simulink library "SPART_Lib"  (R2016b)
settings: Solver=ode45  StartTime=0.0  StopTime=10.0  RelTol=1e-3  EnableMultiTasking=on
undefined symbols (not defined in the file): n, Newton, q00, q0dot0, qm0, Raphson, robot, T_Ln_EE
libraries: SPART_Lib x3, dspinverses x1
settings Model: Creator=Josep  LastModifiedBy=Josep
settings DataIOCC: LimitDataPoints=on  SaveFormat=Array
settings OptimizationCC: LifeSpan=inf
settings DebuggingCC: AllowSymbolicDim=off  SFUnexpectedBacktrackingDiag=warning  SFNoUnconditionalDefaultTransitionDiag=warning  SFExecutionAtInitializationDiag=none
settings HardwareCC: ProdBitPerPointer=32  ProdBitPerSizeT=32  ProdBitPerPtrDiffT=32  ProdLargestAtomicFloat=None  ProdIntDivRoundTo=Undefined  ProdEndianess=Unspecified  ProdWordSize=32  ProdHWDeviceType=32-bit Generic
settings ModelReferenceCC: PropagateSignalLabelsOutOfModel=off
settings GRTTargetCC: TargetLangStandard=C89/C90 (ANSI)  GeneratePreprocessorConditionals=Disable all
settings ConfigComp: CovMetricSettings=dw  CovHtmlReporting=on  CovSaveCumulativeToWorkspaceVar=on  CovSaveSingleToWorkspaceVar=on  CovExternalEMLEnable=off

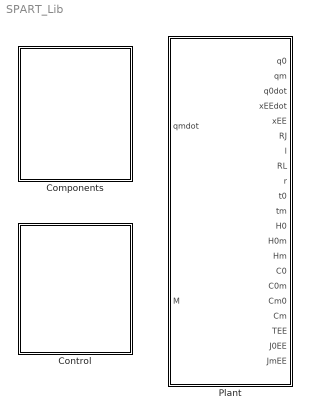
== system SPART_Lib ==
  Components : Subsystem
  Control : Subsystem
  Plant : Subsystem  TreatAsAtomicUnit=on
      settings: MinAlgLoopOccurrences=on

== system SPART_Lib/Components ==
  Base Reaction : Subsystem
  EndEffector : Subsystem
  Jstar : Subsystem
  Matrices : Subsystem

== system SPART_Lib/Control ==
  Base Control : Subsystem
  Desired-Reaction-Maneuver : Subsystem  mask{xdot_I=[1:6], q0dot_I=[1:6]}
      mask prompts: xdot_I "xdot - Indices"; q0dot_I "q0dot - Indices"
      mask help: Desired-Reaction-Maneuver
      settings: MinAlgLoopOccurrences=on
  "Resolved-Motion-Rate " : Subsystem
      settings: MinAlgLoopOccurrences=on
  Resolved-Motion-Rate Minimize Floating Kinematic Energy : Subsystem
      settings: MinAlgLoopOccurrences=on

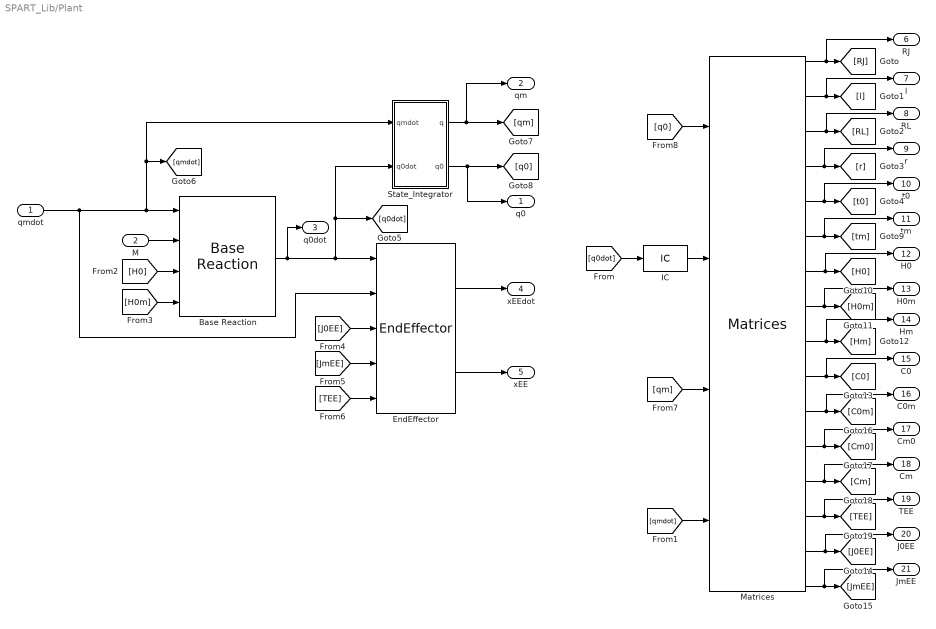
== system SPART_Lib/Plant ==
  qmdot : Inport
  M : Inport  Port=2
  Base Reaction : SPART_Lib/Components/Base Reaction
  EndEffector : SPART_Lib/Components/EndEffector
  IC : InitialCondition  Value=q0dot0
  Matrices : SPART_Lib/Components/Matrices
  State_Integrator : Subsystem
  "q0 " : Outport
  qm : Outport  Port=2
  "q0dot " : Outport  Port=3
  xEEdot : Outport  Port=4
  xEE : Outport  Port=5
  RJ : Outport  Port=6
  l : Outport  Port=7
  RL : Outport  Port=8
  r : Outport  Port=9
  t0 : Outport  Port=10
  "tm " : Outport  Port=11
  "H0 " : Outport  Port=12
  "H0m " : Outport  Port=13
  "Hm " : Outport  Port=14
  "C0 " : Outport  Port=15
  "C0m " : Outport  Port=16
  "Cm0 " : Outport  Port=17
  "Cm " : Outport  Port=18
  TEE : Outport  Port=19
  "J0EE " : Outport  Port=20
  JmEE : Outport  Port=21
  wires:
  [q0dot] -> IC/1
  IC/1 -> Matrices/2
  [q0] -> Matrices/1
  [qm] -> Matrices/3
  [qmdot] -> Matrices/4
  Matrices/1 -> RJ/1, [RJ]
  [H0] -> Base Reaction/3
  [H0m] -> Base Reaction/4
  [J0EE] -> EndEffector/3
  [JmEE] -> EndEffector/4
  [TEE] -> EndEffector/5
  Base Reaction/1 -> "q0dot "/1, EndEffector/1, State_Integrator/2(q0dot), [q0dot]
  qmdot/1 -> EndEffector/2, Base Reaction/1, [qmdot], State_Integrator/1(qmdot)
  M/1 -> Base Reaction/2
  State_Integrator/1(q) -> qm/1, [qm]
  State_Integrator/2(q0) -> "q0 "/1, [q0]
  Matrices/2 -> l/1, [l]
  Matrices/3 -> [RL], RL/1
  Matrices/4 -> r/1, [r]
  Matrices/5 -> t0/1, [t0]
  EndEffector/2 -> xEE/1
  EndEffector/1 -> xEEdot/1
  Matrices/6 -> "tm "/1, [tm]
  Matrices/7 -> "H0 "/1, [H0]
  Matrices/8 -> "H0m "/1, [H0m]
  Matrices/9 -> "Hm "/1, [Hm]
  Matrices/10 -> "C0 "/1, [C0]
  Matrices/11 -> [C0m], "C0m "/1
  Matrices/12 -> "Cm0 "/1, [Cm0]
  Matrices/13 -> "Cm "/1, [Cm]
  Matrices/14 -> TEE/1, [TEE]
  Matrices/15 -> "J0EE "/1, [J0EE]
  Matrices/16 -> JmEE/1, [JmEE]

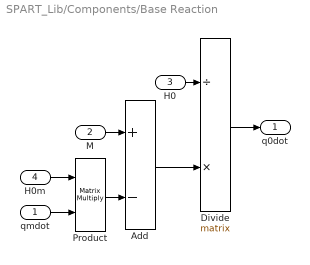
== system SPART_Lib/Components/Base Reaction ==
  qmdot : Inport
  M : Inport  Port=2
  H0 : Inport  Port=3
  H0m : Inport  Port=4
  Add : Sum  Inputs=+-
  Divide : Product  Inputs=/*  Multiplication=Matrix(*)
  Product : Product  Multiplication=Matrix(*)
  q0dot : Outport
  wires:
  Divide/1 -> q0dot/1
  H0/1 -> Divide/1
  M/1 -> Add/1
  Add/1 -> Divide/2
  Product/1 -> Add/2
  H0m/1 -> Product/1
  qmdot/1 -> Product/2

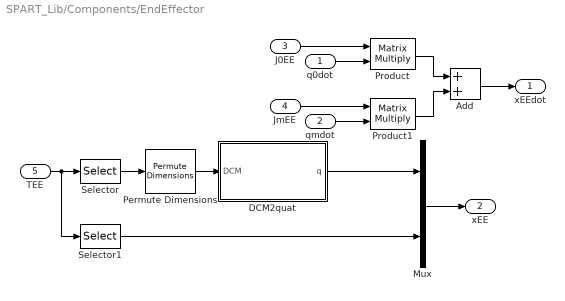
== system SPART_Lib/Components/EndEffector ==
  "q0dot " : Inport
  qmdot : Inport  Port=2
  J0EE : Inport  Port=3
  JmEE : Inport  Port=4
  TEE : Inport  Port=5
  Add : Sum
  DCM2quat : MATLAB Function  TreatAsAtomicUnit=on
  Mux : Mux  Inputs=2
  Permute Dimensions : PermuteDimensions
  Product : Product  Multiplication=Matrix(*)
  Product1 : Product  Multiplication=Matrix(*)
  Selector : Selector  NumberOfDimensions=2  InputPortWidth=6  IndexOptions=Index vector (dialog),Index vector (dialog)  Indices=[1:3],[1:3]  OutputSizes=1,1
  Selector1 : Selector  NumberOfDimensions=2  InputPortWidth=6  IndexOptions=Index vector (dialog),Index vector (dialog)  Indices=[1:3],[4]  OutputSizes=1,1
  xEEdot : Outport
  xEE : Outport  Port=2
  wires:
  Product/1 -> Add/1
  Product1/1 -> Add/2
  Add/1 -> xEEdot/1
  "q0dot "/1 -> Product/2
  qmdot/1 -> Product1/2
  Mux/1 -> xEE/1
  J0EE/1 -> Product/1
  JmEE/1 -> Product1/1
  DCM2quat/1(q) -> Mux/1
  Selector/1 -> Permute Dimensions/1
  TEE/1 -> Selector/1, Selector1/1
  Selector1/1 -> Mux/2
  Permute Dimensions/1 -> DCM2quat/1(DCM)

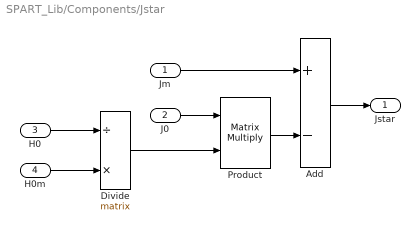
== system SPART_Lib/Components/Jstar ==
  "Jm " : Inport
  J0 : Inport  Port=2
  H0 : Inport  Port=3
  H0m : Inport  Port=4
  Add : Sum  Inputs=+-
  Divide : Product  Inputs=/*  Multiplication=Matrix(*)
  Product : Product  Multiplication=Matrix(*)
  Jstar : Outport
  wires:
  H0m/1 -> Divide/2
  Add/1 -> Jstar/1
  J0/1 -> Product/1
  Divide/1 -> Product/2
  H0/1 -> Divide/1
  Product/1 -> Add/2
  "Jm "/1 -> Add/1

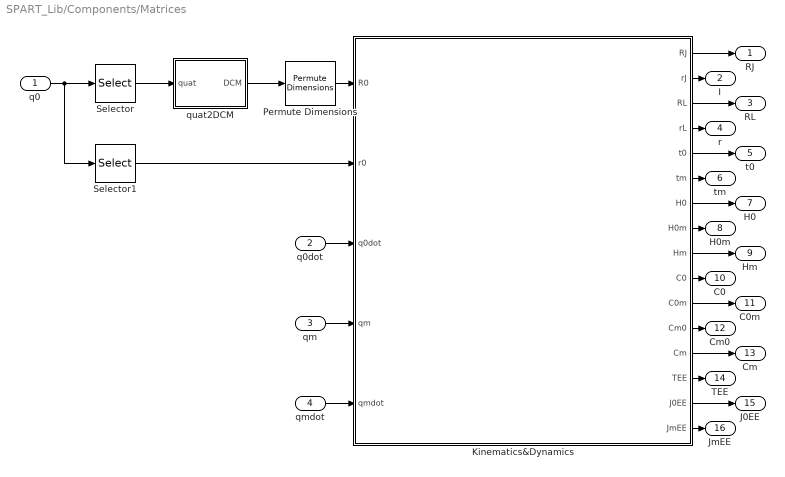
== system SPART_Lib/Components/Matrices ==
  q0 : Inport
  "q0dot " : Inport  Port=2
  qm : Inport  Port=3
  qmdot : Inport  Port=4
  Kinematics&Dynamics : MATLAB Function  TreatAsAtomicUnit=on
  Permute Dimensions : PermuteDimensions
  Selector : Selector  InputPortWidth=7  IndexOptions=Index vector (dialog)  Indices=[1:4]  OutputSizes=1
  Selector1 : Selector  InputPortWidth=7  IndexOptions=Index vector (dialog)  Indices=[5:7]  OutputSizes=1
  quat2DCM : MATLAB Function  TreatAsAtomicUnit=on
  RJ : Outport
  I : Outport  Port=2
  RL : Outport  Port=3
  r : Outport  Port=4
  t0 : Outport  Port=5
  tm : Outport  Port=6
  H0 : Outport  Port=7
  H0m : Outport  Port=8
  Hm : Outport  Port=9
  C0 : Outport  Port=10
  C0m : Outport  Port=11
  Cm0 : Outport  Port=12
  Cm : Outport  Port=13
  TEE : Outport  Port=14
  J0EE : Outport  Port=15
  JmEE : Outport  Port=16
  wires:
  Kinematics&Dynamics/1(RJ) -> RJ/1
  Kinematics&Dynamics/2(rJ) -> I/1
  Kinematics&Dynamics/3(RL) -> RL/1
  Kinematics&Dynamics/4(rL) -> r/1
  Kinematics&Dynamics/5(t0) -> t0/1
  q0/1 -> Selector/1, Selector1/1
  quat2DCM/1(DCM) -> Permute Dimensions/1
  Selector/1 -> quat2DCM/1(quat)
  Kinematics&Dynamics/6(tm) -> tm/1
  Kinematics&Dynamics/7(H0) -> H0/1
  Kinematics&Dynamics/9(Hm) -> Hm/1
  Selector1/1 -> Kinematics&Dynamics/2(r0)
  Permute Dimensions/1 -> Kinematics&Dynamics/1(R0)
  "q0dot "/1 -> Kinematics&Dynamics/3(q0dot)
  qm/1 -> Kinematics&Dynamics/4(qm)
  qmdot/1 -> Kinematics&Dynamics/5(qmdot)
  Kinematics&Dynamics/8(H0m) -> H0m/1
  Kinematics&Dynamics/10(C0) -> C0/1
  Kinematics&Dynamics/12(Cm0) -> Cm0/1
  Kinematics&Dynamics/15(J0EE) -> J0EE/1
  Kinematics&Dynamics/11(C0m) -> C0m/1
  Kinematics&Dynamics/13(Cm) -> Cm/1
  Kinematics&Dynamics/16(JmEE) -> JmEE/1
  Kinematics&Dynamics/14(TEE) -> TEE/1

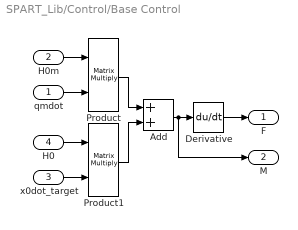
== system SPART_Lib/Control/Base Control ==
  qmdot : Inport
  H0m : Inport  Port=2
  x0dot_target : Inport  Port=3
  H0 : Inport  Port=4
  Add : Sum
  Derivative : Derivative
  Product : Product  Multiplication=Matrix(*)
  Product1 : Product  Multiplication=Matrix(*)
  F : Outport
  M : Outport  Port=2
  wires:
  H0m/1 -> Product/1
  qmdot/1 -> Product/2
  Add/1 -> M/1, Derivative/1
  Product/1 -> Add/1
  Product1/1 -> Add/2
  H0/1 -> Product1/1
  x0dot_target/1 -> Product1/2
  Derivative/1 -> F/1

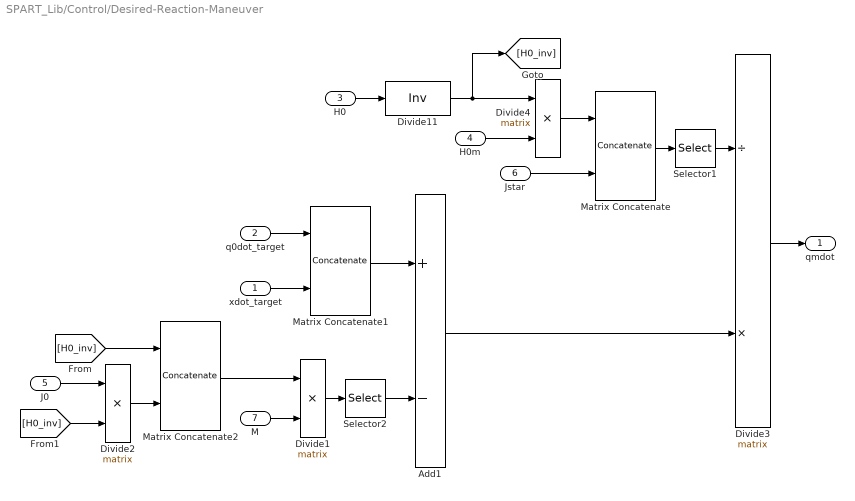
== system SPART_Lib/Control/Desired-Reaction-Maneuver ==
  xdot_target : Inport
  q0dot_target : Inport  Port=2
  H0 : Inport  Port=3
  H0m : Inport  Port=4
  J0 : Inport  Port=5
  Jstar : Inport  Port=6
  M : Inport  Port=7
  Add1 : Sum  Inputs=+-
  Divide1 : Product  Inputs=**  Multiplication=Matrix(*)
  Divide11 : Product  Inputs=/  Multiplication=Matrix(*)
  Divide2 : Product  Inputs=**  Multiplication=Matrix(*)
  Divide3 : Product  Inputs=/*  Multiplication=Matrix(*)
  Divide4 : Product  Inputs=**  Multiplication=Matrix(*)
  Matrix Concatenate : Concatenate  Mode=Multidimensional array
  Matrix Concatenate1 : Concatenate  Mode=Multidimensional array
  Matrix Concatenate2 : Concatenate  Mode=Multidimensional array
  Selector1 : Selector  NumberOfDimensions=2  InputPortWidth=3  IndexOptions=Index vector (dialog),Select all  Indices=[q0dot_I,5+xdot_I],[1:n]  OutputSizes=1,1
  Selector2 : Selector  NumberOfDimensions=2  InputPortWidth=3  IndexOptions=Index vector (dialog),Index vector (dialog)  Indices=[q0dot_I,5+xdot_I],[1]  OutputSizes=1,1
  qmdot : Outport
  wires:
  Divide3/1 -> qmdot/1
  Matrix Concatenate/1 -> Selector1/1
  Divide4/1 -> Matrix Concatenate/1
  H0m/1 -> Divide4/2
  Jstar/1 -> Matrix Concatenate/2
  xdot_target/1 -> Matrix Concatenate1/2
  q0dot_target/1 -> Matrix Concatenate1/1
  Matrix Concatenate1/1 -> Add1/1
  H0/1 -> Divide11/1
  Divide11/1 -> [H0_inv], Divide4/1
  [H0_inv] -> Matrix Concatenate2/1
  Matrix Concatenate2/1 -> Divide1/1
  M/1 -> Divide1/2
  Divide1/1 -> Selector2/1
  Divide2/1 -> Matrix Concatenate2/2
  J0/1 -> Divide2/1
  [H0_inv] -> Divide2/2
  Add1/1 -> Divide3/2
  Selector2/1 -> Add1/2
  Selector1/1 -> Divide3/1

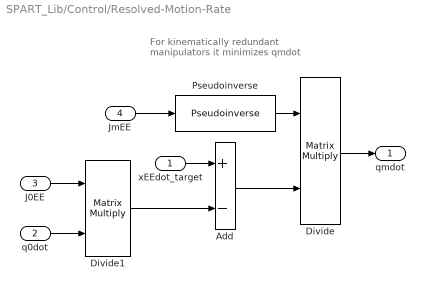
== system SPART_Lib/Control/Resolved-Motion-Rate  ==
  note: For kinematically redundant manipulators it minimizes qmdot
  xEEdot_target : Inport
  q0dot : Inport  Port=2
  J0EE : Inport  Port=3
  JmEE : Inport  Port=4
  Add : Sum  Inputs=+-
  Divide : Product  Inputs=**  Multiplication=Matrix(*)
  Divide1 : Product  Inputs=**  Multiplication=Matrix(*)
  Pseudoinverse : dspinverses/Pseudoinverse  wanterr=off
  qmdot : Outport
  wires:
  Divide/1 -> qmdot/1
  Add/1 -> Divide/2
  Divide1/1 -> Add/2
  J0EE/1 -> Divide1/1
  Pseudoinverse/1 -> Divide/1
  JmEE/1 -> Pseudoinverse/1
  q0dot/1 -> Divide1/2
  xEEdot_target/1 -> Add/1

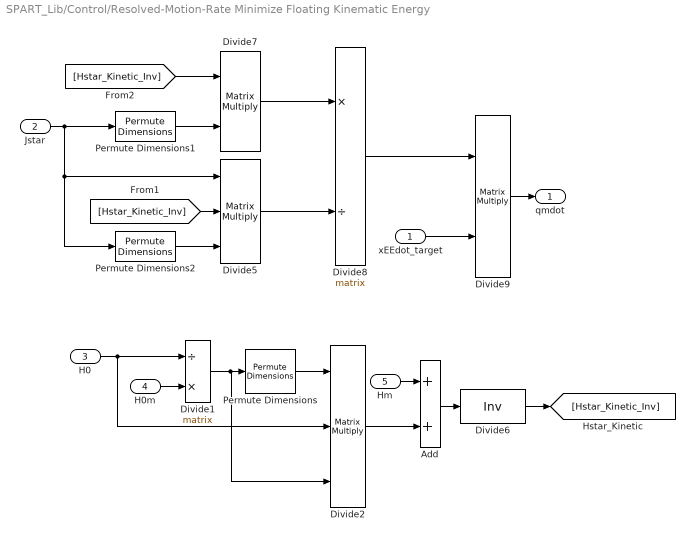
== system SPART_Lib/Control/Resolved-Motion-Rate Minimize Floating Kinematic Energy ==
  xEEdot_target : Inport
  Jstar : Inport  Port=2
  H0 : Inport  Port=3
  H0m : Inport  Port=4
  Hm : Inport  Port=5
  Add : Sum
  Divide1 : Product  Inputs=/*  Multiplication=Matrix(*)
  Divide2 : Product  Inputs=***  Multiplication=Matrix(*)
  Divide5 : Product  Inputs=***  Multiplication=Matrix(*)
  Divide6 : Product  Inputs=/  Multiplication=Matrix(*)
  Divide7 : Product  Inputs=**  Multiplication=Matrix(*)
  Divide8 : Product  Inputs=*/  Multiplication=Matrix(*)
  Divide9 : Product  Inputs=**  Multiplication=Matrix(*)
  Permute Dimensions : PermuteDimensions
  Permute Dimensions1 : PermuteDimensions
  Permute Dimensions2 : PermuteDimensions
  qmdot : Outport
  wires:
  Divide6/1 -> [Hstar_Kinetic_Inv]
  Divide5/1 -> Divide8/2
  Divide9/1 -> qmdot/1
  Divide8/1 -> Divide9/1
  Divide7/1 -> Divide8/1
  Jstar/1 -> Permute Dimensions1/1, Permute Dimensions2/1, Divide5/1
  H0m/1 -> Divide1/2
  Permute Dimensions/1 -> Divide2/1
  Divide1/1 -> Divide2/3, Permute Dimensions/1
  H0/1 -> Divide2/2, Divide1/1
  Divide2/1 -> Add/2
  Hm/1 -> Add/1
  xEEdot_target/1 -> Divide9/2
  [Hstar_Kinetic_Inv] -> Divide7/1
  Permute Dimensions1/1 -> Divide7/2
  [Hstar_Kinetic_Inv] -> Divide5/2
  Add/1 -> Divide6/1
  Permute Dimensions2/1 -> Divide5/3

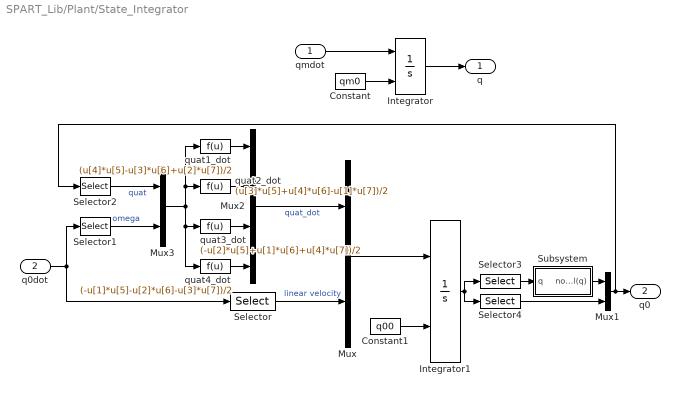
== system SPART_Lib/Plant/State_Integrator ==
  qmdot : Inport
  q0dot : Inport  Port=2
  Constant : Constant  Value=qm0
  Constant1 : Constant  Value=q00
  Integrator : Integrator  InitialConditionSource=external
  Integrator1 : Integrator  InitialConditionSource=external
  Mux : Mux  Inputs=2
  Mux1 : Mux  Inputs=2
  Mux2 : Mux
  Mux3 : Mux  Inputs=2
  Selector : Selector  InputPortWidth=6  IndexOptions=Index vector (dialog)  Indices=[4:6]  OutputSizes=1
  Selector1 : Selector  InputPortWidth=6  IndexOptions=Index vector (dialog)  Indices=[1:3]  OutputSizes=1
  Selector2 : Selector  InputPortWidth=7  IndexOptions=Index vector (dialog)  Indices=[1:4]  OutputSizes=1
  Selector3 : Selector  InputPortWidth=7  IndexOptions=Index vector (dialog)  Indices=[1:4]  OutputSizes=1
  Selector4 : Selector  InputPortWidth=7  IndexOptions=Index vector (dialog)  Indices=[5:7]  OutputSizes=1
  Subsystem : Subsystem
  quat1_dot : Fcn  Expr=(u[4]*u[5]-u[3]*u[6]+u[2]*u[7])/2
  quat2_dot : Fcn  Expr=(u[3]*u[5]+u[4]*u[6]-u[1]*u[7])/2
  quat3_dot : Fcn  Expr=(-u[2]*u[5]+u[1]*u[6]+u[4]*u[7])/2
  quat4_dot : Fcn  Expr=(-u[1]*u[5]-u[2]*u[6]-u[3]*u[7])/2
  q : Outport
  q0 : Outport  Port=2
  wires:
  Integrator/1 -> q/1
  qmdot/1 -> Integrator/1
  Constant/1 -> Integrator/2
  Constant1/1 -> Integrator1/2
  Mux/1 -> Integrator1/1
  Mux2/1 -> Mux/1  "quat_dot"
  Selector/1 -> Mux/2  "linear velocity"
  q0dot/1 -> Selector/1, Selector1/1
  Mux1/1 -> Selector2/1, q0/1
  Selector1/1 -> Mux3/2  "omega"
  Subsystem/1(normal(q)) -> Mux1/1
  Integrator1/1 -> Selector4/1, Selector3/1
  Selector3/1 -> Subsystem/1(q)
  Selector4/1 -> Mux1/2
  Mux3/1 -> quat4_dot/1, quat3_dot/1, quat1_dot/1, quat2_dot/1
  quat1_dot/1 -> Mux2/1
  quat2_dot/1 -> Mux2/2
  quat3_dot/1 -> Mux2/3
  quat4_dot/1 -> Mux2/4
  Selector2/1 -> Mux3/1  "quat"

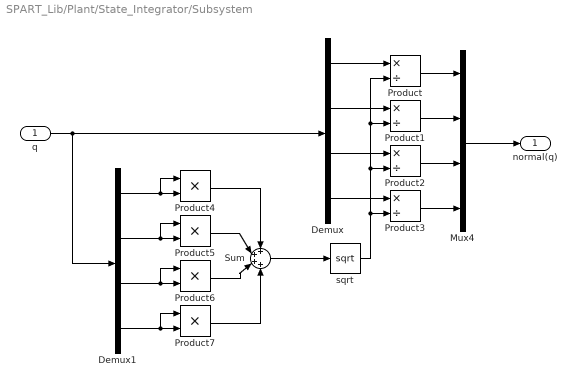
== system SPART_Lib/Plant/State_Integrator/Subsystem ==
  q : Inport
  Demux : Demux
  Demux1 : Demux
  Mux4 : Mux
  Product{,1..3} (4 alike) : Product  Inputs=*/
  Product{4..7} (4 alike) : Product
  Sum : Sum  Inputs=4
  sqrt : Sqrt  AlgorithmType=Newton-Raphson  SaturateOnIntegerOverflow=on
  normal(q) : Outport
  wires:
  Product3/1 -> Mux4/4
  Product2/1 -> Mux4/3
  Product1/1 -> Mux4/2
  Product/1 -> Mux4/1
  sqrt/1 -> Product3/2, Product2/2, Product/2, Product1/2
  Mux4/1 -> normal(q)/1
  Demux/3 -> Product2/1
  Demux/1 -> Product/1
  Demux/2 -> Product1/1
  Demux/4 -> Product3/1
  Demux1/4 -> Product7/1, Product7/2
  Demux1/3 -> Product6/1, Product6/2
  Demux1/2 -> Product5/1, Product5/2
  Demux1/1 -> Product4/1, Product4/2
  Product7/1 -> Sum/4
  Product6/1 -> Sum/3
  Product5/1 -> Sum/2
  Product4/1 -> Sum/1
  Sum/1 -> sqrt/1
  q/1 -> Demux1/1, Demux/1

== matlab function SPART_Lib/Components/Matrices/Kinematics&Dynamics ==
  data: RJ output; rJ output; RL output; rL output; t0 output; tm output; H0 output; H0m output; Hm output; R0 input; r0 input; q0dot input; qm input; qmdot input; robot parameter; C0 output; C0m output; Cm0 output; Cm output; TEE output; J0EE output; JmEE output; T_Ln_EE parameter
function [RJ,rJ,RL,rL,t0,tm,H0,H0m,Hm,C0,C0m,Cm0,Cm,TEE,J0EE,JmEE] = Kinematics_Dynamics(R0,r0,q0dot,qm,qmdot,robot,T_Ln_EE)


%Kinematics
[RJ,RL,rJ,rL,e,g]=Kinematics(R0,r0,qm,robot);
%End-Effector
TEE=[RL(1:3,1:3,end),rL(1:3,end);zeros(1,3),1]*T_Ln_EE;
%Differential Kinematics
[Bij,Bi0,P0,pm]=DiffKinematics(R0,r0,rL,e,g,robot);
%Velocities
[t0,tm]=Velocities(Bij,Bi0,P0,pm,q0dot,qmdot,robot);
%Inertias
[I0,Im]=I_I(R0,RL,robot);
%Mass Composite Body matrix
[M0_tilde,Mm_tilde]=MCB(I0,Im,Bij,Bi0,robot);
%Generalized Inertia matrix
[H0, H0m, Hm] = GIM(M0_tilde,Mm_tilde,Bij,Bi0,P0,pm,robot);
%Generalized Convective Inertia matrix
[C0, C0m, Cm0, Cm] = CIM(t0,tm,I0,Im,M0_tilde,Mm_tilde,Bij,Bi0,P0,pm,robot);
%End-effector Jacobian
[J0EE, JmEE]=Jacob(TEE(1:3,4),r0,rL,P0,pm,robot.n_links_joints,robot);



end

== matlab function SPART_Lib/Components/Matrices/quat2DCM ==
  data: quat input; DCM output
function DCM = quat2DCM(quat)
%Converts quaternion to a DCM
%
%Uses the functions under the Utilities folder

DCM=quat_DCM(quat);

end

== matlab function SPART_Lib/Components/EndEffector/DCM2quat ==
  data: DCM input; q output
function q = DCM2quat(DCM)
%Convert Direction Cosine Matrix (DCM) to quaterion q
%
%Uses the functions under the Utilities folder


q=DCM_quat(DCM);

end
